simulink model "modBF"  (R2021a)
settings: Solver=VariableStepAuto  StartTime=0.0  StopTime=3600  FixedStep=1  MaxStep=10  RelTol=1e-3
libraries: pid_lib x2
settings Model: Creator=F73736  LastModifiedBy=F73736

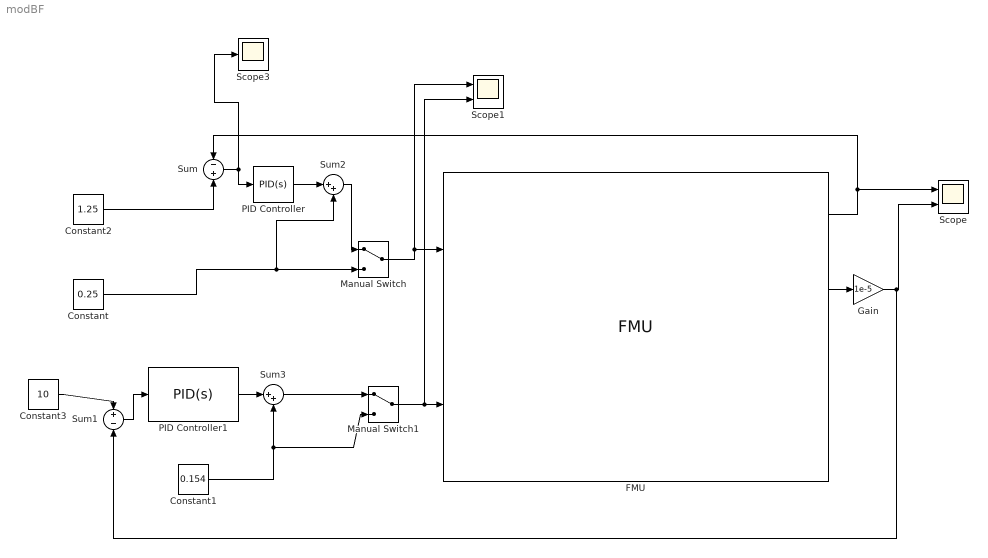
== system modBF ==
  Constant : Constant  Value=0.25
  Constant1 : Constant  Value=0.154  VectorParams1D=off
  Constant2 : Constant  Value=1.25
  Constant3 : Constant  Value=10
  FMU : FMU  FMUName=Dimensionnement_chaudiere.fmu  FMUMode=CoSimulation  genericCombustion=struct('kcham',1,'Acham',1,'Xpth',0.01,'ImbCV',0,'ImbBF',0,'Cpcd',500,'Tbf',500,'Xbf',0.1)  fuelSourcePQ=struct('P0',100000.0,'Q0',0.141329,'T0',300,'LHV',48000000.0,'Cp',1000.0,'Hum',0.0,'Xc',0.75,'Xh',0.25,'Xo',0,'Xn',0,'Xs',0,'Xashes',0,'Vol',0,'rho',0.72)  sourcePQ=struct('P0',110000,'Q0',0.049241,'h0',104928)  sourcePQ1=struct('P0',110000,'Q0',2.50943,'T0',300,'Xco2',0.0006,'Xh2o',0,'Xo2',0.2314,'Xso2',0)  constante10=struct('k',1067930.0)  constante2=struct('k',2.78)  constante8=struct('k',2580000.0)  sinkQ1=struct('Q0',2.78,'h0',2580000.0)  sourceP=struct('P0',300000,'T0',290,'h0',100000,'mode',int32(1))  heatExchangerWall=struct('L',8,'D',0.05,'e',0.003,'lambda',21.4,'cpw',573,'rhow',4579,'T0',350,'ntubes',1400)  staticWallFlueGasesExchanger=struct('NbTub',int32(1400),'DPc',0,'L',8,'Dext',0.05,'step_L',0.033,'step_T',0.066,'St',100,'Encras',1.0,'Fa',0.7,'Tp0',471.06,'CSailettes',1,'Coeff',1)  controlValve=struct('option_interpolation',int32(1),'fluid',int32(1),'mode',int32(0))  dynamicDrumAdapt=struct('R',1.25,'L',8,'Vf0',0.5,'P0',1000000,'Ccond',0.01,'Cevap',0.13,'Xlo',0,'Xvo',0.9975,'Kvl',1000,'Klp',400,'Kvp',100,'Kpa',0,'Mp',117000.0,'cpp',600,'NbTub',int32(1400),'L1',8,'PasT',0.023,'Dext',0.056,'DIc',1.4,'PasL',0.06,'Lc',2.5,'COPl',1)  constante3=struct('k',723029)  gain1=struct('Gain',20.687)  mask(Dimensionnement_chaudiere_fmu [Co-Simulation, v2.0]){}
      mask Display:
      | disp('Dimensionnement_chaudiere_fmu');
      | port_label('output',1,'Niv');
      | port_label('output',2,'pv');
      | port_label('output',3,'CPUtime');
      | port_label('output',4,'EventCounter');
      | port_label('input',1,'Ouv');
      | port_label('input',2,'Qfuel');
  Gain : Gain  Gain=1e-5
  Manual Switch : ManualSwitch
  Manual Switch1 : ManualSwitch
  PID Controller : pid_lib/PID Controller  Controller=PID  Form=Ideal  TimeDomain=Continuous-time  UseExternalTs=off  SampleTime=-1  IntegratorMethod=Forward Euler  FilterMethod=Forward Euler  ControllerParametersSource=internal  P=20  I=1/200  D=0  UseFilter=on  N=100  TunerSelectOption=Transfer Function Based (PID Tuner App)  InitialConditionSource=internal  InitialConditionForIntegrator=0  InitialConditionForFilter=0  DifferentiatorICPrevScaledInput=0  ExternalReset=none  TrackingMode=off  Kt=1  LimitOutput=off  SatLimitsSource=internal  UpperSaturationLimit=inf  LowerSaturationLimit=-inf  LinearizeAsGain=on  AntiWindupMode=none  Kb=1  POutMin=[]  POutMax=[]  IOutMin=[]  IOutMax=[]  DOutMin=[]  DOutMax=[]  NOutMin=[]  NOutMax=[]  SumOutMin=[]  SumOutMax=[]  SaturationOutMin=[]  SaturationOutMax=[]  PParamMin=[]  PParamMax=[]  IParamMin=[]  IParamMax=[]  DParamMin=[]  DParamMax=[]  NParamMin=[]  NParamMax=[]  KbParamMin=[]  KbParamMax=[]  KtParamMin=[]  KtParamMax=[]  KbOutMin=[]  KbOutMax=[]  KtOutMin=[]  KtOutMax=[]  IntegratorOutMin=[]  IntegratorOutMax=[]  FilterOutMin=[]  FilterOutMax=[]  SumI1OutMin=[]  SumI1OutMax=[]  SumI2OutMin=[]  SumI2OutMax=[]  SumI3OutMin=[]  SumI3OutMax=[]  SumI4OutMin=[]  SumI4OutMax=[]  SumDOutMin=[]  SumDOutMax=[]  DifferentiatorOutMin=[]  DifferentiatorOutMax=[]  FilterDiffOutCoefMin=[]  FilterDiffOutCoefMax=[]  ReciprocalOutMin=[]  ReciprocalOutMax=[]  SumDenOutMin=[]  SumDenOutMax=[]  SumNumOutMin=[]  SumNumOutMax=[]  DivideOutMin=[]  DivideOutMax=[]  UdiffTsProdOutMin=[]  UdiffTsProdOutMax=[]  NTsProdOutMin=[]  NTsProdOutMax=[]  UintegralTsProdOutMin=[]  UintegralTsProdOutMax=[]  UngainTsProdOutMin=[]  UngainTsProdOutMax=[]  IntegratorContinuousStateAttributes=''  IntegratorStateMustResolveToSignalObject=off  IntegratorRTWStateStorageClass=Auto  FilterContinuousStateAttributes=''  FilterStateMustResolveToSignalObject=off  FilterRTWStateStorageClass=Auto  ParallelPVariant=Passthrough  IdealPVariant=InternalParameters  IVariant=InternalParameters  DVariant=InternalParameters  IntegratorVariant=Continuous  SatVariant=Disabled  AWVariant=Passthrough  PCopyVariant=Disabled  TRVariant=Disabled  FdbkBlocksVariant=Forward  IdealPFdbkVariant=Disabled  SatFdbkVariant=Disabled  DerivativeFilterVariant=ContFilter  NVariant=InternalParameters  NCopyVariant=Disabled  FilterICVariant=InternalICsFilter  IntegratorICVariant=InternalICs  ExternalResetVariant=Disabled  TRSumVariant=Passthrough  SumFdbkVariant=Disabled  SumVariant=Sum_PID  TsampFilterVariant=InternalTs  TsampNgainVariant=Passthrough  TsampIntegralVariant=Passthrough  ExternalSaturationOutDataTypeStr=Inherit: Same as second input
  PID Controller1 : pid_lib/PID Controller  Controller=PID  Form=Ideal  TimeDomain=Continuous-time  UseExternalTs=off  SampleTime=-1  IntegratorMethod=Forward Euler  FilterMethod=Forward Euler  ControllerParametersSource=internal  P=0.03  I=1/500  D=0  UseFilter=on  N=100  TunerSelectOption=Transfer Function Based (PID Tuner App)  ZeroCross=off  InitialConditionSource=internal  InitialConditionForIntegrator=0  InitialConditionForFilter=0  DifferentiatorICPrevScaledInput=0  ExternalReset=none  TrackingMode=off  Kt=1  LimitOutput=off  SatLimitsSource=internal  UpperSaturationLimit=inf  LowerSaturationLimit=-inf  LinearizeAsGain=on  AntiWindupMode=none  Kb=1  POutMin=[]  POutMax=[]  IOutMin=[]  IOutMax=[]  DOutMin=[]  DOutMax=[]  NOutMin=[]  NOutMax=[]  SumOutMin=[]  SumOutMax=[]  SaturationOutMin=[]  SaturationOutMax=[]  PParamMin=[]  PParamMax=[]  IParamMin=[]  IParamMax=[]  DParamMin=[]  DParamMax=[]  NParamMin=[]  NParamMax=[]  KbParamMin=[]  KbParamMax=[]  KtParamMin=[]  KtParamMax=[]  KbOutMin=[]  KbOutMax=[]  KtOutMin=[]  KtOutMax=[]  IntegratorOutMin=[]  IntegratorOutMax=[]  FilterOutMin=[]  FilterOutMax=[]  SumI1OutMin=[]  SumI1OutMax=[]  SumI2OutMin=[]  SumI2OutMax=[]  SumI3OutMin=[]  SumI3OutMax=[]  SumI4OutMin=[]  SumI4OutMax=[]  SumDOutMin=[]  SumDOutMax=[]  DifferentiatorOutMin=[]  DifferentiatorOutMax=[]  FilterDiffOutCoefMin=[]  FilterDiffOutCoefMax=[]  ReciprocalOutMin=[]  ReciprocalOutMax=[]  SumDenOutMin=[]  SumDenOutMax=[]  SumNumOutMin=[]  SumNumOutMax=[]  DivideOutMin=[]  DivideOutMax=[]  UdiffTsProdOutMin=[]  UdiffTsProdOutMax=[]  NTsProdOutMin=[]  NTsProdOutMax=[]  UintegralTsProdOutMin=[]  UintegralTsProdOutMax=[]  UngainTsProdOutMin=[]  UngainTsProdOutMax=[]  IntegratorContinuousStateAttributes=''  IntegratorStateMustResolveToSignalObject=off  IntegratorRTWStateStorageClass=Auto  FilterContinuousStateAttributes=''  FilterStateMustResolveToSignalObject=off  FilterRTWStateStorageClass=Auto  ParallelPVariant=Passthrough  IdealPVariant=InternalParameters  IVariant=InternalParameters  DVariant=InternalParameters  IntegratorVariant=Continuous  SatVariant=Disabled  AWVariant=Passthrough  PCopyVariant=Disabled  TRVariant=Disabled  FdbkBlocksVariant=Forward  IdealPFdbkVariant=Disabled  SatFdbkVariant=Disabled  DerivativeFilterVariant=ContFilter  NVariant=InternalParameters  NCopyVariant=Disabled  FilterICVariant=InternalICsFilter  IntegratorICVariant=InternalICs  ExternalResetVariant=Disabled  TRSumVariant=Passthrough  SumFdbkVariant=Disabled  SumVariant=Sum_PID  TsampFilterVariant=InternalTs  TsampNgainVariant=Passthrough  TsampIntegralVariant=Passthrough  ExternalSaturationOutDataTypeStr=Inherit: Same as second input
  Scope : Scope  NumInputPorts=2
  Scope1 : Scope  NumInputPorts=2
  Scope3 : Scope
  Sum : Sum  Inputs=-+
  Sum1 : Sum  Inputs=+-
  Sum2 : Sum  Inputs=|++
  Sum3 : Sum  Inputs=|++
  wires:
  FMU/1 -> Scope/1, Sum/1
  FMU/2 -> Gain/1
  Constant2/1 -> Sum/2
  Sum/1 -> Scope3/1, PID Controller/1
  Constant/1 -> Sum2/2, Manual Switch/2
  Manual Switch/1 -> Scope1/1, FMU/1
  Gain/1 -> Sum1/2, Scope/2
  Constant1/1 -> Sum3/2, Manual Switch1/2
  Constant3/1 -> Sum1/1
  Sum1/1 -> PID Controller1/1
  Manual Switch1/1 -> Scope1/2, FMU/2
  PID Controller/1 -> Sum2/1
  Sum2/1 -> Manual Switch/1
  PID Controller1/1 -> Sum3/1
  Sum3/1 -> Manual Switch1/1
